simulink model "AutomatedVehicle_Simulink"  (R2020b)
settings: Solver=ode3  StartTime=0.0  StopTime=150  FixedStep=Td  RelTol=1e-3
values from neighbouring files (symbols this model uses):
  Td = 0.05    [ControlLaw_MPC_SS.m]    (also in Initialization_MPC_SS.m)
libraries: simulink x1
settings Model: Creator=asierzubizarreta  LastModifiedBy=snopv
settings DataIOCC: LimitDataPoints=on  SaveFormat=Array  ReturnWorkspaceOutputs=off
settings OptimizationCC: BlockReduction=off  BooleanDataType=off  LifeSpan=inf
settings DebuggingCC: SaveWithParameterizedLinksMsg=none  UnderspecifiedInitializationDetection=Classic  MergeDetectMultiDrivingBlocksExec=none  SignalResolutionControl=TryResolveAllWithWarning  SFUnexpectedBacktrackingDiag=warning  SFNoUnconditionalDefaultTransitionDiag=warning  SFExecutionAtInitializationDiag=none  ArithmeticOperatorsInVariantConditions=warning
settings HardwareCC: ProdBitPerPointer=32  ProdBitPerSizeT=32  ProdBitPerPtrDiffT=32  ProdLargestAtomicFloat=None  ProdIntDivRoundTo=Undefined  ProdEndianess=Unspecified  ProdWordSize=32  ProdHWDeviceType=32-bit Generic  TargetUnknown=on
settings ModelReferenceCC: PropagateSignalLabelsOutOfModel=off
settings SFSimCC: SimUseLocalCustomCode=off  CustomCodeUndefinedFunction=UseInterfaceOnly
settings RTWCC: RTWUseLocalCustomCode=off
settings CodeAppCC: StateflowObjectComments=on
settings GRTTargetCC: TargetLangStandard=C89/C90 (ANSI)
settings ConfigComp: CovMetricSettings=dw  CovSaveCumulativeToWorkspaceVar=on  CovSaveSingleToWorkspaceVar=on  CovExternalEMLEnable=off

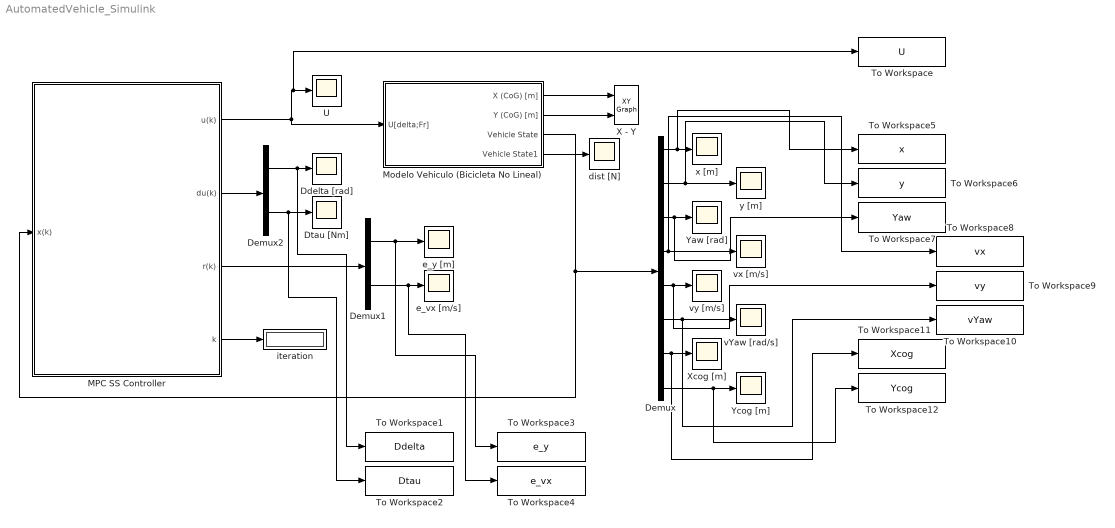
== system AutomatedVehicle_Simulink ==
  Ddelta [rad] : Scope
  Demux : Demux  Outputs=8
  Demux1 : Demux  Outputs=2
  Demux2 : Demux  Outputs=2
  Dtau [Nm] : Scope
  MPC SS Controller : Subsystem  TreatAsAtomicUnit=on  SystemSampleTime=Td  mask{PlotCheck=on, Xlim=100}
      mask prompts: PlotCheck "Plotear trayectoria"; Xlim "Tamaño Visor [m]"
      mask init:
      | [parameters, trackdata,Td]=Initialization_MPC_SS;
      | [ny,nx]=size(parameters.C);
      | [nx,nu]=size(parameters.B);
      mask DialogControl DescGroupVar Prompt: MPC Controller
      mask Display:
      | fprintf('MPC SS Control\n\n\n');
      | 
      | 
      | port_label('output',1,'u(k)');
      | port_label('output',2,'du(k)');
      | port_label('output',3,'e(k)');
      | port_label('output',4,'k');
      | port_label('input',1,'x(k)');
  Modelo Vehiculo (Bicicleta No Lineal) : Subsystem  mask(Vehicle Model (nonlinear)){don=off, disturbancetime=1, disturbancevalue=1000}
      mask prompts: don "Disturbance ON"; disturbancetime "Disturbance time (s)"; disturbancevalue "Disturbance Value [N]"
      mask help: Modelo vehículo
      mask init:
      | [parameters, trackdata,Td]=Initialization_MPC_SS;
      | V0=trackdata.V(1);
      mask DialogControl Container3 Prompt: Disturbance
      mask Display:
      | if(ispc==1)
      | 
      |     Filepath=[cd '\ext_G7C_deg01.jpg'];
      | else
      |     Filepath=[cd '/ext_G7C_deg01.jpg'];
      | end
      |     image(Filepath);
  To Workspace : ToWorkspace  VariableName=U  SaveFormat=Timeseries  SampleTime=-1
  To Workspace1 : ToWorkspace  VariableName=Ddelta  SaveFormat=Timeseries  SampleTime=-1
  To Workspace10 : ToWorkspace  VariableName=vYaw  SaveFormat=Timeseries  SampleTime=-1
  To Workspace11 : ToWorkspace  VariableName=Xcog  SaveFormat=Timeseries  SampleTime=-1
  To Workspace12 : ToWorkspace  VariableName=Ycog  SaveFormat=Timeseries  SampleTime=-1
  To Workspace2 : ToWorkspace  VariableName=Dtau  SaveFormat=Timeseries  SampleTime=-1
  To Workspace3 : ToWorkspace  VariableName=e_y  SaveFormat=Timeseries  SampleTime=-1
  To Workspace4 : ToWorkspace  VariableName=e_vx  SaveFormat=Timeseries  SampleTime=-1
  To Workspace5 : ToWorkspace  VariableName=x  SaveFormat=Timeseries  SampleTime=-1
  To Workspace6 : ToWorkspace  VariableName=y  SaveFormat=Timeseries  SampleTime=-1
  To Workspace7 : ToWorkspace  VariableName=Yaw  SaveFormat=Timeseries  SampleTime=-1
  To Workspace8 : ToWorkspace  VariableName=vx  SaveFormat=Timeseries  SampleTime=-1
  To Workspace9 : ToWorkspace  VariableName=vy  SaveFormat=Timeseries  SampleTime=-1
  U : Scope
  X - Y : simulink/Sinks/XY Graph  xmin=-10  xmax=800  ymin=-100  ymax=100  st=-1
  Xcog [m] : Scope
  Yaw [rad] : Scope
  Ycog [m] : Scope
  dist [N] : Scope
  e_vx [m/s] : Scope
  e_y [m] : Scope
  iteration : Display
  vYaw [rad/s] : Scope
  vx [m/s] : Scope
  vy [m/s] : Scope
  x [m] : Scope
  y [m] : Scope
  wires:
  MPC SS Controller/4(k) -> iteration/1
  Modelo Vehiculo (Bicicleta No Lineal)/3(Vehicle State) -> MPC SS Controller/1(x(k)), Demux/1
  MPC SS Controller/1(u(k)) -> To Workspace/1, U/1, Modelo Vehiculo (Bicicleta No Lineal)/1(U[delta;Fr])
  Modelo Vehiculo (Bicicleta No Lineal)/1(X (CoG) [m]) -> X - Y/1
  Modelo Vehiculo (Bicicleta No Lineal)/2(Y (CoG) [m]) -> X - Y/2
  Demux/1 -> To Workspace5/1, x [m]/1
  Demux/2 -> y [m]/1, To Workspace6/1
  Demux/3 -> To Workspace7/1, Yaw [rad]/1
  Demux/5 -> To Workspace9/1, vy [m/s]/1
  Demux/4 -> vx [m/s]/1, To Workspace8/1
  Demux/6 -> vYaw [rad/s]/1, To Workspace10/1
  Demux/7 -> To Workspace11/1, Xcog [m]/1
  Demux/8 -> To Workspace12/1, Ycog [m]/1
  MPC SS Controller/3(r(k)) -> Demux1/1
  Demux1/2 -> To Workspace4/1, e_vx [m/s]/1
  MPC SS Controller/2(du(k)) -> Demux2/1
  Demux2/1 -> To Workspace1/1, Ddelta [rad]/1
  Demux1/1 -> To Workspace3/1, e_y [m]/1
  Modelo Vehiculo (Bicicleta No Lineal)/4(Vehicle State1) -> dist [N]/1
  Demux2/2 -> To Workspace2/1, Dtau [Nm]/1

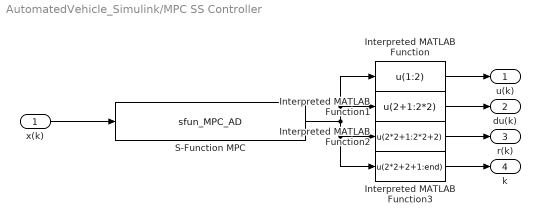
== system AutomatedVehicle_Simulink/MPC SS Controller ==
  x(k) : Inport
  Interpreted MATLAB Function : MATLABFcn  MATLABFcn=u(1:2)  OutputDimensions=2
  Interpreted MATLAB Function1 : MATLABFcn  MATLABFcn=u(2+1:2*2)  OutputDimensions=2
  Interpreted MATLAB Function2 : MATLABFcn  MATLABFcn=u(2*2+1:2*2+2)  OutputDimensions=2
  Interpreted MATLAB Function3 : MATLABFcn  MATLABFcn=u(2*2+2+1:end)  OutputDimensions=1
  S-Function MPC : S-Function  FunctionName=sfun_MPC_AD  Parameters=PlotCheck,Xlim  SFunctionModules=s  SFunctionDeploymentMode=off  EnableBusSupport=off
  u(k) : Outport
  du(k) : Outport  Port=2
  r(k) : Outport  Port=3
  k : Outport  Port=4
  wires:
  Interpreted MATLAB Function3/1 -> k/1
  x(k)/1 -> S-Function MPC/1
  S-Function MPC/1 -> Interpreted MATLAB Function1/1, Interpreted MATLAB Function/1, Interpreted MATLAB Function3/1, Interpreted MATLAB Function2/1
  Interpreted MATLAB Function/1 -> u(k)/1
  Interpreted MATLAB Function1/1 -> du(k)/1
  Interpreted MATLAB Function2/1 -> r(k)/1

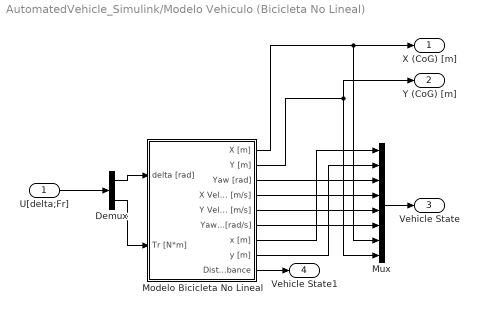
== system AutomatedVehicle_Simulink/Modelo Vehiculo (Bicicleta No Lineal) ==
  U[delta;Fr] : Inport
  Demux : Demux  Outputs=2
  Modelo Bicicleta No Lineal : Subsystem
  Mux : Mux  Inputs=8
  X (CoG) [m] : Outport
  Y (CoG) [m] : Outport  Port=2
  Vehicle State : Outport  Port=3
  Vehicle State1 : Outport  Port=4
  wires:
  Modelo Bicicleta No Lineal/3(Yaw [rad]) -> Mux/3
  Modelo Bicicleta No Lineal/5(Y Velocity [m/s]) -> Mux/5
  Modelo Bicicleta No Lineal/4(X Velocity [m/s]) -> Mux/4
  Modelo Bicicleta No Lineal/6(Yaw Rate [rad/s]) -> Mux/6
  Modelo Bicicleta No Lineal/2(Y [m]) -> Y (CoG) [m]/1, Mux/8
  Demux/2 -> Modelo Bicicleta No Lineal/2(Tr [N*m])
  U[delta;Fr]/1 -> Demux/1
  Demux/1 -> Modelo Bicicleta No Lineal/1(delta [rad])
  Mux/1 -> Vehicle State/1
  Modelo Bicicleta No Lineal/7(x [m]) -> Mux/1
  Modelo Bicicleta No Lineal/8(y [m]) -> Mux/2
  Modelo Bicicleta No Lineal/1(X [m]) -> Mux/7, X (CoG) [m]/1
  Modelo Bicicleta No Lineal/9(Disturbance) -> Vehicle State1/1

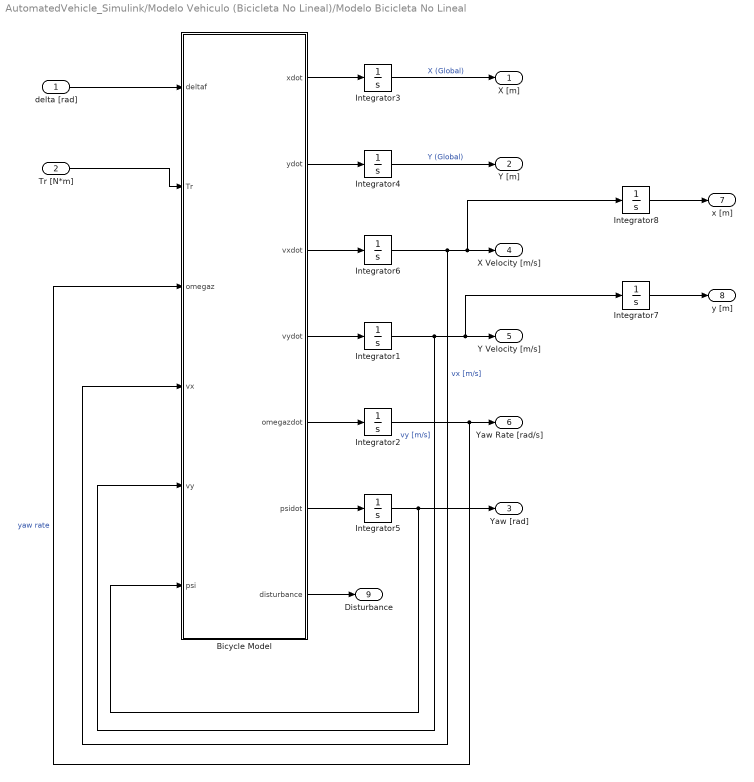
== system AutomatedVehicle_Simulink/Modelo Vehiculo (Bicicleta No Lineal)/Modelo Bicicleta No Lineal ==
  delta [rad] : Inport
  Tr [N*m] : Inport  Port=2
  Bicycle Model : Subsystem
  Integrator{1..5,7..8} (7 alike) : Integrator
  Integrator6 : Integrator  InitialCondition=V0
  X [m] : Outport
  Y [m] : Outport  Port=2
  Yaw [rad] : Outport  Port=3
  X Velocity [m/s] : Outport  Port=4
  Y Velocity [m/s] : Outport  Port=5
  Yaw Rate [rad/s] : Outport  Port=6
  x [m] : Outport  Port=7
  y [m] : Outport  Port=8
  Disturbance : Outport  Port=9
  wires:
  Integrator4/1 -> Y [m]/1  "Y (Global)"
  Integrator2/1 -> Yaw Rate [rad/s]/1, Bicycle Model/3(omegaz)  "yaw rate"
  Bicycle Model/2(ydot) -> Integrator4/1
  delta [rad]/1 -> Bicycle Model/1(deltaf)
  Bicycle Model/1(xdot) -> Integrator3/1
  Integrator3/1 -> X [m]/1  "X (Global)"
  Tr [N*m]/1 -> Bicycle Model/2(Tr)
  Integrator5/1 -> Yaw [rad]/1, Bicycle Model/6(psi)
  Integrator6/1 -> Bicycle Model/4(vx), Integrator8/1, X Velocity [m/s]/1  "vx [m/s]"
  Bicycle Model/3(vxdot) -> Integrator6/1
  Integrator1/1 -> Integrator7/1, Y Velocity [m/s]/1, Bicycle Model/5(vy)  "vy [m/s]"
  Bicycle Model/4(vydot) -> Integrator1/1
  Bicycle Model/5(omegazdot) -> Integrator2/1
  Bicycle Model/6(psidot) -> Integrator5/1
  Integrator7/1 -> y [m]/1
  Integrator8/1 -> x [m]/1
  Bicycle Model/7(disturbance) -> Disturbance/1

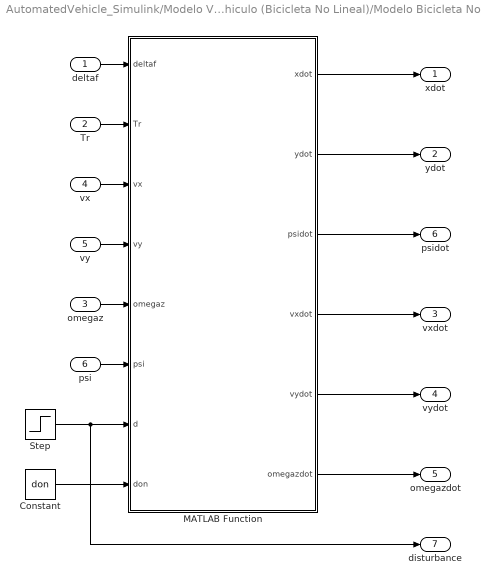
== system AutomatedVehicle_Simulink/Modelo Vehiculo (Bicicleta No Lineal)/Modelo Bicicleta No Lineal/Bicycle Model ==
  deltaf : Inport
  Tr : Inport  Port=2
  omegaz : Inport  Port=3
  vx : Inport  Port=4
  vy : Inport  Port=5
  psi : Inport  Port=6
  Constant : Constant  Value=don
  MATLAB Function : MATLAB Function  TreatAsAtomicUnit=on
  Step : Step  Time=disturbancetime  After=disturbancevalue  SampleTime=0
  xdot : Outport
  ydot : Outport  Port=2
  vxdot : Outport  Port=3
  vydot : Outport  Port=4
  omegazdot : Outport  Port=5
  psidot : Outport  Port=6
  disturbance : Outport  Port=7
  wires:
  deltaf/1 -> MATLAB Function/1(deltaf)
  omegaz/1 -> MATLAB Function/5(omegaz)
  Tr/1 -> MATLAB Function/2(Tr)
  vx/1 -> MATLAB Function/3(vx)
  vy/1 -> MATLAB Function/4(vy)
  psi/1 -> MATLAB Function/6(psi)
  MATLAB Function/1(xdot) -> xdot/1
  MATLAB Function/2(ydot) -> ydot/1
  MATLAB Function/3(psidot) -> psidot/1
  MATLAB Function/4(vxdot) -> vxdot/1
  MATLAB Function/5(vydot) -> vydot/1
  MATLAB Function/6(omegazdot) -> omegazdot/1
  Step/1 -> disturbance/1, MATLAB Function/7(d)
  Constant/1 -> MATLAB Function/8(don)

== matlab function AutomatedVehicle_Simulink/Modelo Vehiculo (Bicicleta No Lineal)/Modelo Bicicleta No Lineal/Bicycle Model/MATLAB Function ==
  data: xdot output; ydot output; psidot output; vxdot output; vydot output; deltaf input; Tr input; vx input; vy input; omegaz input; psi input; omegazdot output; d input; don input
function [xdot,ydot,psidot,vxdot,vydot,omegazdot] = fcn(deltaf,Tr,vx,vy,omegaz,psi,d,don)

%% Parametros Twizy
a = 0.9269;         % [m]  
b = 0.7591;         % [m]
m = 611.5;          % [kg]
Rf = 0.265;         % [m]
Rr = 0.281;         % [m]
Iz = 430.166;       % [kg*m^2]
froll = 0.002;      % [-]
Cr = 42550.81/1.8;  % [N/rad]
Cf = 352.54/2;      % [N/rad]
g = 9.81;
   
alphaf = deltaf - atan((vy+a*omegaz)/vx);  if isnan(alphaf), alphaf = 0; end;
alphar = - atan((vy-b*omegaz)/vx);         if isnan(alphar), alphar = 0; end;

% Angulos pequeños
% alphaf = deltaf - ((vy+a*omegaz)/vx);    if isnan(alphaf), alphaf = 0; end;
% alphar = - ((vy-b*omegaz)/vx);           if isnan(alphar), alphar = 0; end;

Flf = 0;
Flr = Tr/Rr;

Fcf = Cf*alphaf;     % Slip Angles calculados
Fcr = Cr*alphar;

Fxf = Flf*cos(deltaf) - Fcf*sin(deltaf); 
Fxr = Flr;
Fyf = Flf*sin(deltaf) + Fcf*cos(deltaf);
Fyr = Fcr;

if(don==1)
    d=d;
else
    d=0;
    end

AccX = (2*Fxf + 2*Fxr - froll*vx*m*g-d) / m; % x Velocity
AccY = (2*Fyf + 2*Fyr) / m; % y Velocity
omegazdot = (2*a*Fyf - 2*b*Fyr) / Iz; % Yaw Rate

vxdot = AccX + vy*omegaz;
vydot = AccY - vx*omegaz;

xdot = vx*cos(psi) - vy*sin(psi); % x Position (Absolute)
ydot = vx*sin(psi) + vy*cos(psi); % y Position (Absolute)
psidot = omegaz;
